simulink model "progetto3Tenzo"  (Simulink 7.9)
settings: Solver=ode45  StartTime=0.0  StopTime=30  RelTol=1e-3
values from neighbouring files (symbols this model uses):
  AMI = AK1    [AstaTenzo.m]
  AMin = [ ... (first row only)    [AstaTenzo.m]    (also in RiduzioneModello.m = [ 0 1 0 0 0 0 0 0; RiduzioneModello1_05.m = [ 0 1 0 0 0 0 0 0; RiduzioneModello1_10.m = [ 0 1 0 0 0 0 0 0; RiduzioneModello1_15.m)
  Aoss = AMin-V*ClocalMin    [AstaTenzo.m]    (also in RiduzioneModello1_05.m; RiduzioneModello1_10.m; RiduzioneModello1_15.m)
  BMI = BK1    [AstaTenzo.m]
  Bmod = [M BMin]    [AstaTenzo.m]
  Boss = [BMin-V*D V M-V*N]    [AstaTenzo.m]    (also in RiduzioneModello1_05.m = [BMin-V*D V]; RiduzioneModello1_10.m = [BMin-V*D V]; RiduzioneModello1_15.m = [BMin-V*D V])
  ClocalMin = [ ... (first row only)    [AstaTenzo.m]    (also in RiduzioneModello.m; RiduzioneModello1_05.m; RiduzioneModello1_10.m; RiduzioneModello1_15.m)
  CMI = eye(q*mu)    [AstaTenzo.m]
  Coss = eye(n)    [AstaTenzo.m]    (also in RiduzioneModello1_05.m = eye(size(AMin)); RiduzioneModello1_10.m = eye(size(AMin)); RiduzioneModello1_15.m = eye(size(AMin)))
  DMI = zeros(q*mu,q)    [AstaTenzo.m]
  Dmod = [N D]    [AstaTenzo.m]
  Doss = zeros(size(Boss))    [AstaTenzo.m]    (also in RiduzioneModello1_05.m; RiduzioneModello1_10.m; RiduzioneModello1_15.m)
  F1 = F(:,size(AMin,1)+1:size(F,2))    [AstaTenzo.m]
  F2 = F(:,1:size(AMin,1))    [AstaTenzo.m]
  omega = 4    [AstaTenzo.m]    (also in StabilizzazioneRetroazione.m; Tenzo1_10.m)
settings Model: Creator=danilo  LastModifiedBy=userk
settings DebuggingCC: FcnCallInpInsideContextMsg=Use local settings
settings GRTTargetCC: CombineOutputUpdateFcns=off  GRTInterface=on

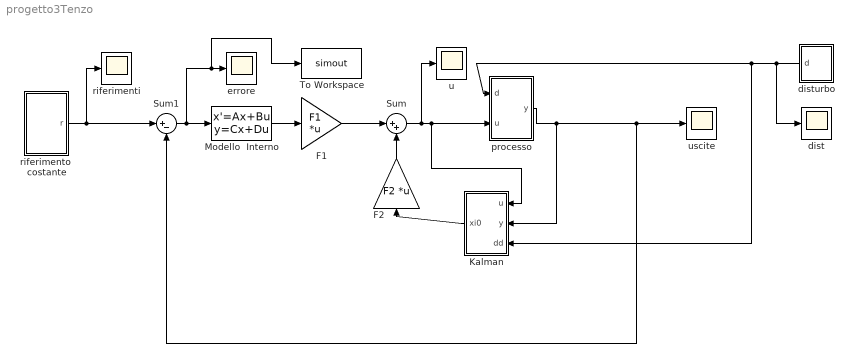
== system progetto3Tenzo ==
  F1 : Gain  Gain=F1  Multiplication=Matrix(K*u) (u vector)
  F2 : Gain  Gain=F2  Multiplication=Matrix(K*u) (u vector)
  Kalman : Subsystem
  Modello  Interno : StateSpace  A=AMI  B=BMI  C=CMI  D=DMI
  Sum : Sum  Inputs=|++
  Sum1 : Sum  Inputs=|+-
  To Workspace : ToWorkspace  VariableName=simout  SampleTime=-1  SaveFormat=Structure
  dist : Scope
      settings: SaveName=ScopeData5
  disturbo : Subsystem
  errore : Scope
      settings: SaveName=ScopeData2
  processo : Subsystem
  riferimenti : Scope
  riferimento  costante : Subsystem
  u : Scope
      settings: SaveName=ScopeData3
  uscite : Scope
      settings: TickLabels=on  YMin=0.75  YMax=4.25
  wires:
  riferimento  costante/1(r) -> Sum1/1, riferimenti/1
  processo/1(y) -> uscite/1, Sum1/2, Kalman/2(y)
  Kalman/1(xi0) -> F2/1
  Modello  Interno/1 -> F1/1
  F2/1 -> Sum/2
  F1/1 -> Sum/1
  Sum/1 -> Kalman/1(u), processo/2(u), u/1
  Sum1/1 -> Modello  Interno/1, errore/1, To Workspace/1
  disturbo/1(d) -> dist/1, processo/1(d), Kalman/3(dd)

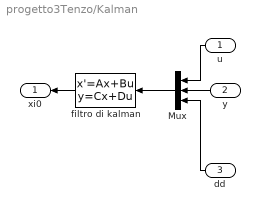
== system progetto3Tenzo/Kalman ==
  u : Inport
  y : Inport  Port=2
  dd : Inport  Port=3
  Mux : Mux  Inputs=[4 4 1]
  filtro di kalman : StateSpace  A=Aoss  B=Boss  C=Coss  D=Doss
  xi0 : Outport
  wires:
  Mux/1 -> filtro di kalman/1
  u/1 -> Mux/1
  filtro di kalman/1 -> xi0/1
  y/1 -> Mux/2
  dd/1 -> Mux/3

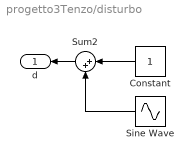
== system progetto3Tenzo/disturbo ==
  Constant : Constant
  Sine Wave : Sin  Frequency=omega  SampleTime=0
  Sum2 : Sum  Inputs=|++
  d : Outport
  wires:
  Sine Wave/1 -> Sum2/2
  Constant/1 -> Sum2/1
  Sum2/1 -> d/1

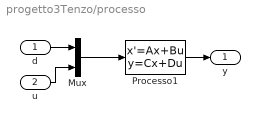
== system progetto3Tenzo/processo ==
  d : Inport
  u : Inport  Port=2
  Mux : Mux  Inputs=[1 4]
  Processo1 : StateSpace  A=AMin  B=Bmod  C=ClocalMin  D=Dmod
  y : Outport
  wires:
  Mux/1 -> Processo1/1
  d/1 -> Mux/1
  Processo1/1 -> y/1
  u/1 -> Mux/2

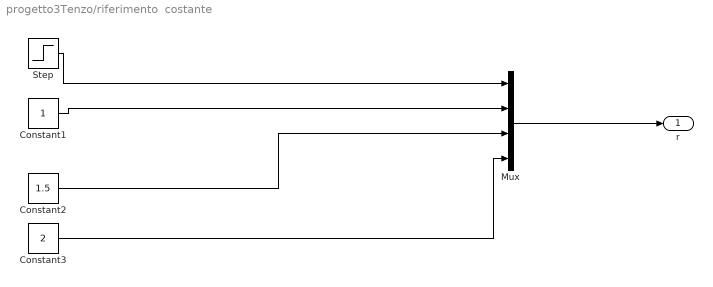
== system progetto3Tenzo/riferimento  costante ==
  Constant1 : Constant
  Constant2 : Constant  Value=1.5
  Constant3 : Constant  Value=2
  Mux : Mux  Inputs=[1 1 1 1]
  Step : Step  Time=3  After=2.5  SampleTime=0
  r : Outport
  wires:
  Mux/1 -> r/1
  Step/1 -> Mux/1
  Constant1/1 -> Mux/2
  Constant2/1 -> Mux/3
  Constant3/1 -> Mux/4
